simulink model "full_vehicle_sim"  (R2025b)
settings: Solver=VariableStepAuto  StartTime=0.0  StopTime=500  RelTol=1e-3
libraries: fl_lib x9, nesl_utility x5, SimscapeFluids_lib x2
(part 1 of 3)
settings Model: Creator=Owner  LastModifiedBy=25han
settings OptimizationCC: ReuseModelBlockBuffer=off
settings RTWCC: GPUComputeCapability=3.5

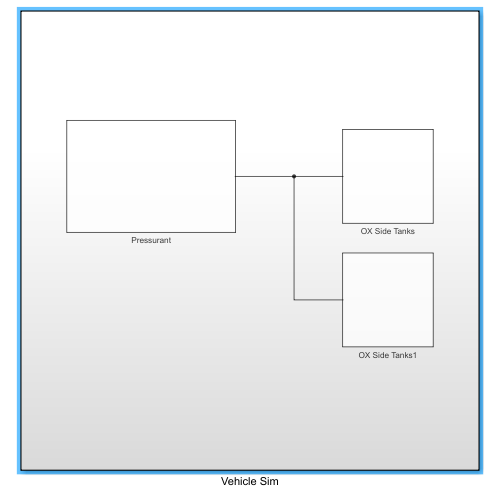
[thumbnail: Simulink's stored preview of the top-level diagram]
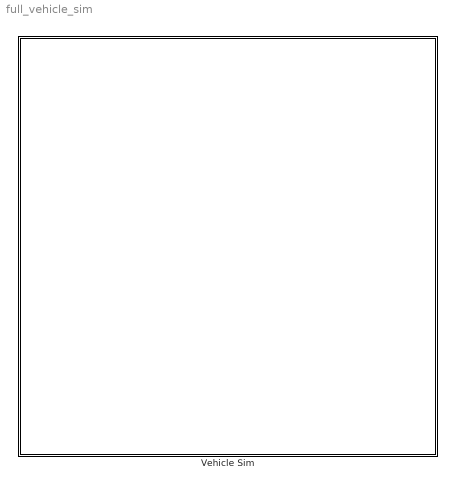
== system full_vehicle_sim ==
  Vehicle Sim : Subsystem

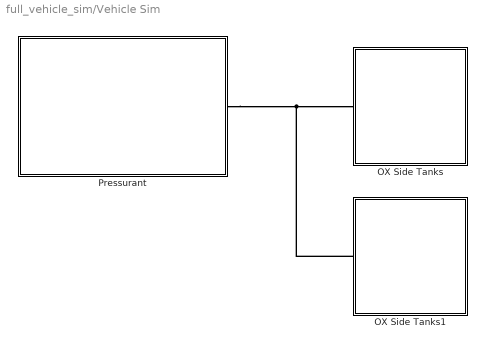
== system full_vehicle_sim/Vehicle Sim ==
  OX Side Tanks : Subsystem
  OX Side Tanks1 : Subsystem
  Pressurant : Subsystem
  connections:
  Pressurant/RConn1 -- OX Side Tanks1/LConn1 -- OX Side Tanks/LConn1

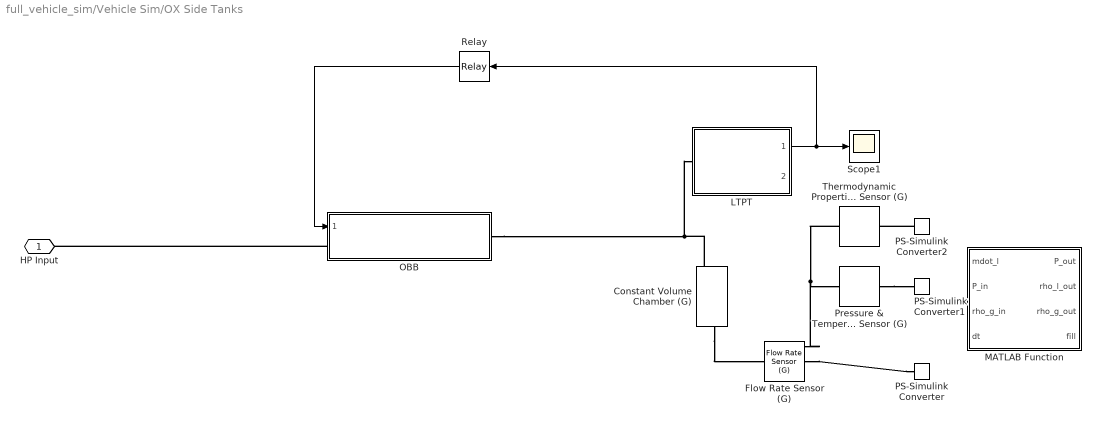
== system full_vehicle_sim/Vehicle Sim/OX Side Tanks ==
  Constant Volume Chamber (G) : fl_lib/Gas/Elements/Constant Volume Chamber (G)  volume=0.01988 m^3  num_ports=foundation.enum.num_ports.two  area_A=0.01 m^2  area_B=0.01 m^2  area_C=0.01 m^2  area_D=0.01 m^2  p_I_specify=on  p_I_priority=High  p_I=500 psi  p_I_nominal_specify=off  p_I_nominal_value=1  p_I_nominal_unit=MPa  T_I_specify=off  T_I_priority=High  T_I=293.15 K  T_I_nominal_specify=off  T_I_nominal_value=1  T_I_nominal_unit=K  rho_I_specify=off  rho_I_priority=None  rho_I=1.2 kg/m^3  rho_I_nominal_specify=off  rho_I_nominal_value=1  rho_I_nominal_unit=kg/m^3
      settings: InternalSimscapePortConfiguration="{\"Bottom\":[],\"Left\":[{\"id\":\"A\",\"label\":\"A\",\"type\":\"foundation.gas.gas\"},{\"id\":\"H\",\"label\":\"H\",\"type\":\"foundation.thermal.thermal\"}],\"Right\":[{\"id\":\"B\",\"label\":\"B\",\"type\":\"foundation.gas.gas\"}],\"Top\":[]}"
  Flow Rate Sensor (G) : fl_lib/Gas/Sensors/Flow Rate Sensor (G)  mass_flow_measure=true  volumetric_flow_measure=false  volumetric_flow_conditions=foundation.enum.volumetric_flow_conditions.actual  p_std=0.101325 MPa  T_std=20 degC  energy_flow_measure=true
      settings: InternalSimscapePortConfiguration="{\"Bottom\":[{\"id\":\"PHI\",\"label\":\"φ\",\"type\":\"output\"}],\"Left\":[{\"id\":\"A\",\"label\":\"A\",\"type\":\"foundation.gas.gas\"}],\"Right\":[{\"id\":\"B\",\"label\":\"B\",\"type\":\"foundation.gas.gas\"},{\"id\":\"M\",\"label\":\"M\",\"type\":\"output\"}],\"Top\":[]}"
  LTPT : Subsystem  ReferencedSubsystem=PT  max_press=5000  lower_val=4  upper_val=20
  MATLAB Function : MATLAB Function  TreatAsAtomicUnit=on
  OBB : Subsystem  ReferencedSubsystem=BangBang
  PS-Simulink Converter : nesl_utility/PS-Simulink Converter  PhysicalDomain=network_engine_domain  SubClassName=ps_output  LeftPortType=input  RightPortType=output  PseudoPeriodic=off  Frequencies=[]  VectorFormat=inherit  Unit=inherit  AffineConversion=off
  PS-Simulink Converter1 : nesl_utility/PS-Simulink Converter  PhysicalDomain=network_engine_domain  SubClassName=ps_output  LeftPortType=input  RightPortType=output  PseudoPeriodic=off  Frequencies=[]  VectorFormat=inherit  Unit=inherit  AffineConversion=off
  PS-Simulink Converter2 : nesl_utility/PS-Simulink Converter  PhysicalDomain=network_engine_domain  SubClassName=ps_output  LeftPortType=input  RightPortType=output  PseudoPeriodic=off  Frequencies=[]  VectorFormat=inherit  Unit=inherit  AffineConversion=off
  Pressure & Temperature Sensor (G) : fl_lib/Gas/Sensors/Pressure & Temperature Sensor (G)  reference=foundation.enum.MeasurementReference.absolute  pressure=true  pressure_spec=foundation.enum.PressureMeasementSpec.Absolute  temperature=false
      settings: InternalSimscapePortConfiguration="{\"Bottom\":[],\"Left\":[{\"id\":\"A\",\"label\":\"A\",\"type\":\"foundation.gas.gas\"}],\"Right\":[{\"id\":\"Pa\",\"label\":\"Pa\",\"type\":\"output\"}],\"Top\":[]}"
  Relay : Relay  OnSwitchValue=501  OffSwitchValue=499  OnOutputValue=0  OffOutputValue=1
  Scope1 : Scope
      settings: ActiveDisplayYMinimum=481.07967715144241  ActiveDisplayYMaximum=554.51912555971307
  Thermodynamic Properties Sensor (G) : fl_lib/Gas/Sensors/Thermodynamic Properties Sensor (G)  enthalpy=false  density=true  specific_heat=false  entropy=false  s_std=3.8635 kJ/(K*kg)  p_std=0.101325 MPa  T_std=293.15 K
      settings: InternalSimscapePortConfiguration="{\"Bottom\":[],\"Left\":[{\"id\":\"A\",\"label\":\"A\",\"type\":\"foundation.gas.gas\"}],\"Right\":[{\"id\":\"RHO\",\"label\":\"ρ\",\"type\":\"output\"}],\"Top\":[]}"
  HP Input : PMIOPort  Side=Left
  wires:
  LTPT/1 -> Relay/1, Scope1/1
  Relay/1 -> OBB/1
  connections:
  OBB/LConn1 -- HP Input/RConn1
  OBB/RConn1 -- Constant Volume Chamber (G)/LConn1 -- LTPT/LConn1
  Constant Volume Chamber (G)/RConn1 -- Flow Rate Sensor (G)/LConn1
  Flow Rate Sensor (G)/RConn1 -- Thermodynamic Properties Sensor (G)/LConn1 -- Pressure & Temperature Sensor (G)/LConn1
  Flow Rate Sensor (G)/RConn2 -- PS-Simulink Converter/LConn1
  Pressure & Temperature Sensor (G)/RConn1 -- PS-Simulink Converter1/LConn1
  PS-Simulink Converter2/LConn1 -- Thermodynamic Properties Sensor (G)/RConn1

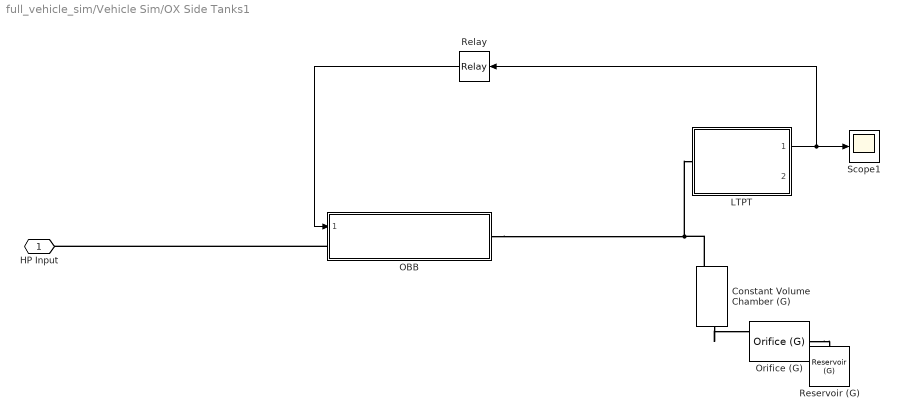
== system full_vehicle_sim/Vehicle Sim/OX Side Tanks1 ==
  Constant Volume Chamber (G) : fl_lib/Gas/Elements/Constant Volume Chamber (G)  volume=0.01988 m^3  num_ports=foundation.enum.num_ports.two  area_A=0.01 m^2  area_B=0.01 m^2  area_C=0.01 m^2  area_D=0.01 m^2  p_I_specify=on  p_I_priority=High  p_I=500 psi  p_I_nominal_specify=off  p_I_nominal_value=1  p_I_nominal_unit=MPa  T_I_specify=off  T_I_priority=High  T_I=293.15 K  T_I_nominal_specify=off  T_I_nominal_value=1  T_I_nominal_unit=K  rho_I_specify=off  rho_I_priority=None  rho_I=1.2 kg/m^3  rho_I_nominal_specify=off  rho_I_nominal_value=1  rho_I_nominal_unit=kg/m^3
      settings: InternalSimscapePortConfiguration="{\"Bottom\":[],\"Left\":[{\"id\":\"A\",\"label\":\"A\",\"type\":\"foundation.gas.gas\"},{\"id\":\"H\",\"label\":\"H\",\"type\":\"foundation.thermal.thermal\"}],\"Right\":[{\"id\":\"B\",\"label\":\"B\",\"type\":\"foundation.gas.gas\"}],\"Top\":[]}"
  LTPT : Subsystem  ReferencedSubsystem=PT  max_press=5000  lower_val=4  upper_val=20
  OBB : Subsystem  ReferencedSubsystem=BangBang
  Orifice (G) : SimscapeFluids_lib/Gas/Valves & Orifices/Orifice (G)  orifice_type=foundation.enum.constant_variable.variable  orifice_parameterization=fluids.gas.valves_orifices.enum.OrificeParameterization.Area  opening_characteristic=fluids.gas.valves_orifices.enum.OpeningCharacteristics.Linear  Cv_constant=4  Cv_max=4  L_Cv_TLU=0 : 0.2 : 1  Cv_TLU=[1e-06, .8, 1.6, 2.4, 3.2, 4]  xT_Cv=0.7  Kv_constant=3.6  Kv_max=3.6  L_Kv_TLU=0 : 0.2 : 1  Kv_TLU=[1e-06, .72, 1.44, 2.16, 2.88, 3.6]  xT_Kv=0.7  C_constant=12 l/(bar*s)  B_crit_constant=0.3  C_max=12 l/(bar*s)  B_crit_linear=0.3  L_C_TLU=0 : 0.2 : 1  C_TLU=[1e-05, 2.4, 4.8, 7.2, 9.6, 12] l/(bar*s)  B_crit_TLU=0.3 * ones(1, 6)  m=0.5  T_ref_C=293.15 K  rho_ref_C=1.185 kg/m^3  orifice_area_constant=1e-4 m^2  orifice_area_max=0.005 m^2  L_orifice_area_TLU=0 : 0.2 : 1  orifice_area_TLU=[1e-10, 2e-05, 4e-05, 6e-05, 8e-05, .0001] m^2  Cd=0.64  leakage_fraction=1e-6  smoothing_factor=0.01  B_lam=0.999  area=0.01 m^2
      settings: InternalSimscapePortConfiguration="{\"Bottom\":[],\"Left\":[{\"id\":\"A\",\"label\":\"A\",\"type\":\"foundation.gas.gas\"},{\"id\":\"L\",\"label\":\"L\",\"type\":\"input\"}],\"Right\":[{\"id\":\"B\",\"label\":\"B\",\"type\":\"foundation.gas.gas\"}],\"Top\":[]}"
  Relay : Relay  OnSwitchValue=501  OffSwitchValue=499  OnOutputValue=0  OffOutputValue=1
  Reservoir (G) : fl_lib/Gas/Elements/Reservoir (G)  pressure_spec=foundation.enum.pressure_spec.atmospheric  reservoir_pressure=0.101325 MPa  reservoir_temperature=293.15 K  area_A=0.01 m^2
  Scope1 : Scope
      settings: ActiveDisplayYMinimum=475.87662602112414  ActiveDisplayYMaximum=610.75660755220383
  HP Input : PMIOPort  Side=Left
  wires:
  LTPT/1 -> Relay/1, Scope1/1
  Relay/1 -> OBB/1
  connections:
  OBB/LConn1 -- HP Input/RConn1
  OBB/RConn1 -- Constant Volume Chamber (G)/LConn1 -- LTPT/LConn1
  Constant Volume Chamber (G)/RConn1 -- Orifice (G)/LConn1
  Orifice (G)/RConn1 -- Reservoir (G)/LConn1
